simulink model "regulated_system"  (R2013a)
settings: Solver=ode45  StartTime=0.0  StopTime=10.0  RelTol=1e-3
undefined symbols (not defined in the file or in its folder): J_mean_1, J_mean_2, K_mean_1, K_mean_2
settings Model: Creator=torbal  LastModifiedBy=torbal

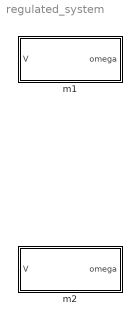
== system regulated_system ==
  m1 : Subsystem
  m2 : Subsystem

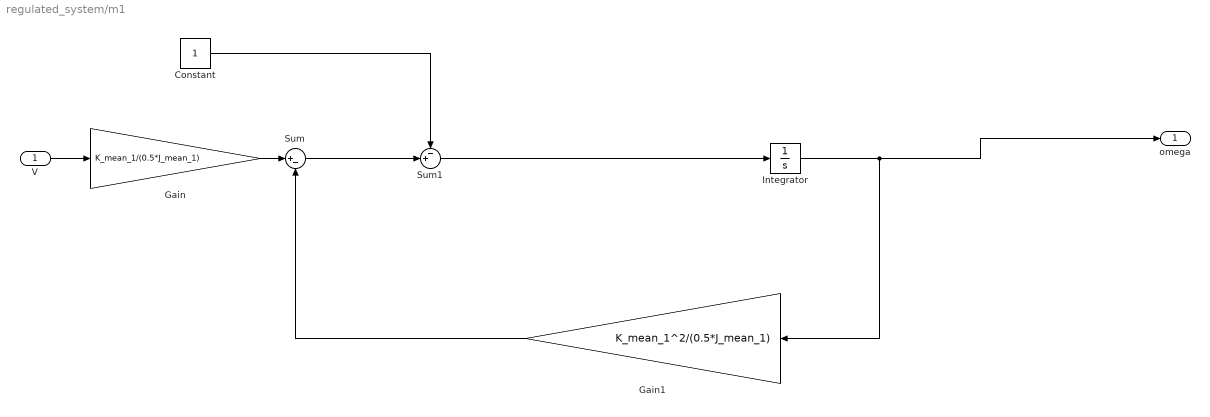
== system regulated_system/m1 ==
  V : Inport
  Constant : Constant
  Gain : Gain  Gain=K_mean_1/(0.5*J_mean_1)
  Gain1 : Gain  Gain=K_mean_1^2/(0.5*J_mean_1)
  Integrator : Integrator
  Sum : Sum  Inputs=|+-
  Sum1 : Sum  Inputs=-+|
  omega : Outport
  wires:
  V/1 -> Gain/1
  Gain/1 -> Sum/1
  Gain1/1 -> Sum/2
  Integrator/1 -> Gain1/1, omega/1
  Sum1/1 -> Integrator/1
  Sum/1 -> Sum1/2
  Constant/1 -> Sum1/1

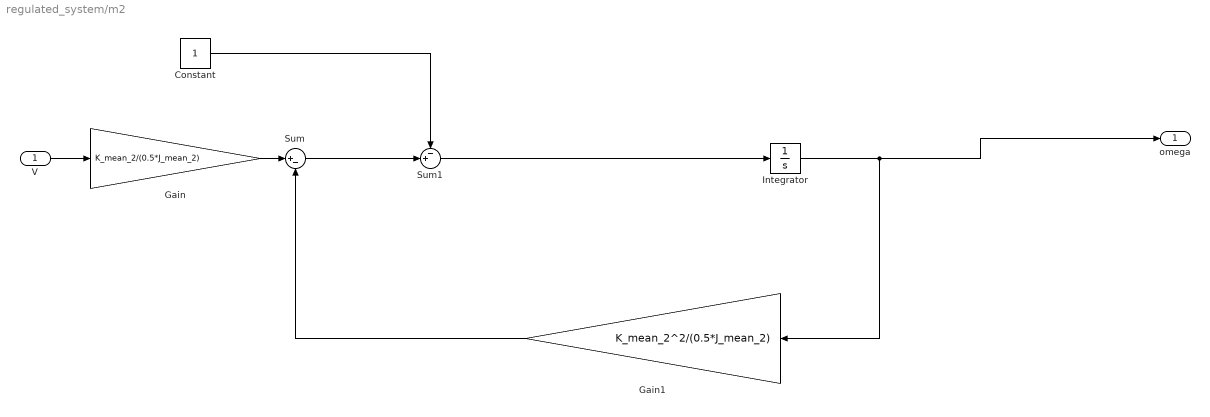
== system regulated_system/m2 ==
  V : Inport
  Constant : Constant
  Gain : Gain  Gain=K_mean_2/(0.5*J_mean_2)
  Gain1 : Gain  Gain=K_mean_2^2/(0.5*J_mean_2)
  Integrator : Integrator
  Sum : Sum  Inputs=|+-
  Sum1 : Sum  Inputs=-+|
  omega : Outport
  wires:
  V/1 -> Gain/1
  Gain/1 -> Sum/1
  Gain1/1 -> Sum/2
  Integrator/1 -> Gain1/1, omega/1
  Sum1/1 -> Integrator/1
  Sum/1 -> Sum1/2
  Constant/1 -> Sum1/1
